simulink model "GUIDANCE_MODEL"  (R2021b)
settings: Solver=FixedStepAuto  StartTime=0  StopTime=10.0  FixedStep=0.2  RelTol=1e-3
settings Model: Creator=verti  LastModifiedBy=verti

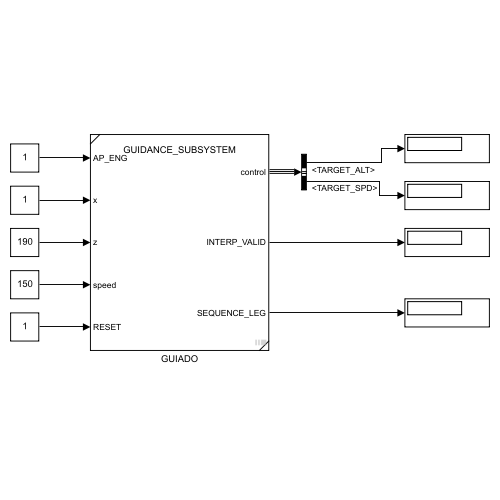
[thumbnail: Simulink's stored preview of the top-level diagram]
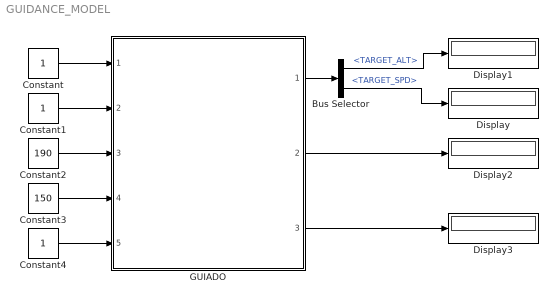
== system GUIDANCE_MODEL ==
  Bus Selector : BusSelector  OutputSignals=TARGET_ALT,TARGET_SPD
  Constant : Constant
  Constant1 : Constant
  Constant2 : Constant  Value=190
  Constant3 : Constant  Value=150
  Constant4 : Constant
  Display{,1..3} (4 alike) : Display
  GUIADO : Subsystem  ReferencedSubsystem=GUIDANCE_SUBSYSTEM
  wires:
  Constant/1 -> GUIADO/1
  Constant1/1 -> GUIADO/2
  Constant3/1 -> GUIADO/4
  Constant2/1 -> GUIADO/3
  GUIADO/1 -> Bus Selector/1
  Bus Selector/1 -> Display1/1  "<TARGET_ALT>"
  Bus Selector/2 -> Display/1  "<TARGET_SPD>"
  Constant4/1 -> GUIADO/5
  GUIADO/2 -> Display2/1
  GUIADO/3 -> Display3/1
